simulink model "mpc_simulation_tracking"  (R2020b)
settings: Solver=VariableStepAuto  StartTime=0.0  StopTime=3  RelTol=1e-3
InitFcn:
  | mpc_example_tracking
values from neighbouring files (symbols this model uses):
  A = [0 0 1 0 0 ... (first row only)    [DesignProjectP2.m]    (also in DesignProjectP3.m; DesignProject_OffsetP3.m; mpc_example_regulation.m = [ 	 0,       0,              1,  0, 0; 	 0,       0,        ; mpc_example_tracking.m = [ 	 0,       0,              1,  0, 0; 	 0,       0,        )
  B = [0;0;0;0;1/La]    [DesignProjectP2.m]    (also in DesignProjectP3.m; DesignProject_OffsetP3.m; mpc_example_regulation.m = [0; 0; 0; 0; 1/La]; mpc_example_tracking.m = [0; 0; 0; 0; 1/La])
  g = 9.81    [DesignProjectP2.m]    (also in DesignProjectP3.m; DesignProject_OffsetP3.m; mpc_example_regulation.m; mpc_example_tracking.m)
  Jl = 0.001    [DesignProjectP2.m]    (also in DesignProjectP3.m; DesignProject_OffsetP3.m; mpc_example_regulation.m; mpc_example_tracking.m)
  l = 0.1    [DesignProjectP2.m]    (also in DesignProjectP3.m; DesignProject_OffsetP3.m; mpc_example_regulation.m; mpc_example_tracking.m)
  m = 0.1    [DesignProjectP2.m]    (also in DesignProjectP3.m; DesignProject_OffsetP3.m; mpc_example_regulation.m; mpc_example_tracking.m)
  mpc_initial_state = mpcstate(mpc_obj)    [mpc_example_regulation.m]    (also in mpc_example_tracking.m)
  sample_time = 1/50    (= 0.02)    [mpc_example_regulation.m]    (also in mpc_example_tracking.m)
libraries: mpclib x1
settings Model: Creator=pbeuchat  LastModifiedBy=pbeuchat

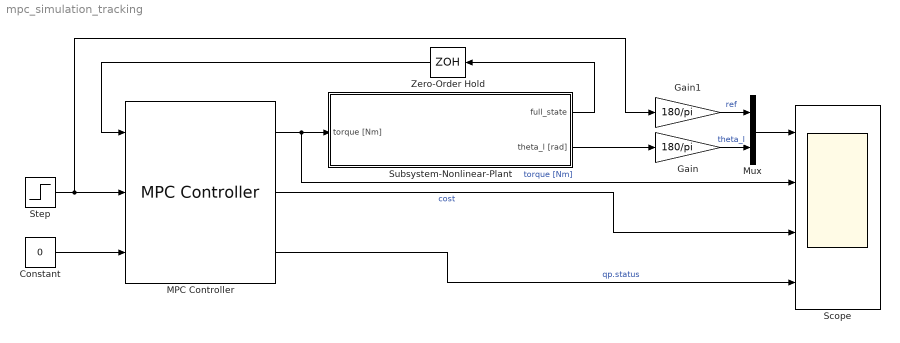
== system mpc_simulation_tracking ==
  Constant : Constant  Value=0
  Gain : Gain  Gain=180/pi
  Gain1 : Gain  Gain=180/pi
  MPC Controller : mpclib/MPC Controller  SCDEnableBlockLinearizationSpecification=on  mpcobj=mpc_obj  x0=mpc_initial_state  is_multiple=0  enable_value=0  return_u0=off  updateMPCinCallerWorkspace=on  md_inport=off  mv_inport=off  uref_inport=on  return_cost=on  return_mvseq=off  return_qpstatus=on  return_xseq=off  return_state=off  return_ovseq=off  state_inport=on  umin_inport=off  umax_inport=off  ymin_inport=off  ymax_inport=off  cc_inport=off  ywt_inport=off  uwt_inport=off  duwt_inport=off  rhoeps_inport=off  pm_inport=off  MaximumP=10  HorizonChoice=FixedHorizon  n_ts=0.02  n_p=20  n_mv=1  n_md=0  n_ud=0  n_mo=1  n_uo=0  BlockDataType=double  SampleTimeInherited=off  switch_inport=off
  Mux : Mux  Inputs=2
  Scope : Scope  NumInputPorts=4
  Step : Step  After=deg2rad(20)  SampleTime=0
  Subsystem-Nonlinear-Plant : Subsystem
  Zero-Order Hold : ZeroOrderHold  SampleTime=sample_time
  wires:
  MPC Controller/1 -> Scope/2, Subsystem-Nonlinear-Plant/1(torque [Nm])  "torque [Nm]"
  Subsystem-Nonlinear-Plant/1(full_state) -> Zero-Order Hold/1
  Step/1 -> Gain1/1, MPC Controller/2
  MPC Controller/2 -> Scope/3  "cost"
  MPC Controller/3 -> Scope/4  "qp.status"
  Constant/1 -> MPC Controller/3
  Subsystem-Nonlinear-Plant/2(theta_l [rad]) -> Gain/1
  Gain/1 -> Mux/2  "theta_l"
  Mux/1 -> Scope/1
  Gain1/1 -> Mux/1  "ref"
  Zero-Order Hold/1 -> MPC Controller/1

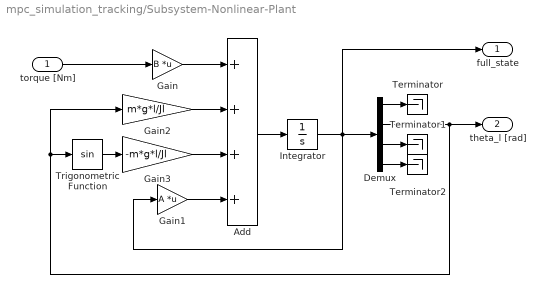
== system mpc_simulation_tracking/Subsystem-Nonlinear-Plant ==
  torque [Nm] : Inport
  Add : Sum  Inputs=++++
  Demux : Demux
  Gain : Gain  Gain=B  Multiplication=Matrix(K*u)
  Gain1 : Gain  Gain=A  Multiplication=Matrix(K*u)
  Gain2 : Gain  Gain=m*g*l/Jl
  Gain3 : Gain  Gain=-m*g*l/Jl
  Integrator : Integrator  InitialCondition=mpc_initial_state.Plant
  Terminator : Terminator
  Terminator1 : Terminator
  Terminator2 : Terminator
  Trigonometric Function : Trigonometry
  full_state : Outport
  theta_l [rad] : Outport  Port=2
  wires:
  Demux/2 -> theta_l [rad]/1, Gain2/1, Trigonometric Function/1
  torque [Nm]/1 -> Gain/1
  Integrator/1 -> full_state/1, Demux/1, Gain1/1
  Demux/1 -> Terminator/1
  Demux/3 -> Terminator1/1
  Demux/4 -> Terminator2/1
  Trigonometric Function/1 -> Gain3/1
  Add/1 -> Integrator/1
  Gain/1 -> Add/1
  Gain1/1 -> Add/4
  Gain2/1 -> Add/2
  Gain3/1 -> Add/3
